simulink model "Lag_Compensator"  (R2023a)
settings: Solver=VariableStepAuto  StartTime=0.0  StopTime=30  RelTol=1e-3
settings Model: Creator=zhouwenjie  LastModifiedBy=zhouwenjie

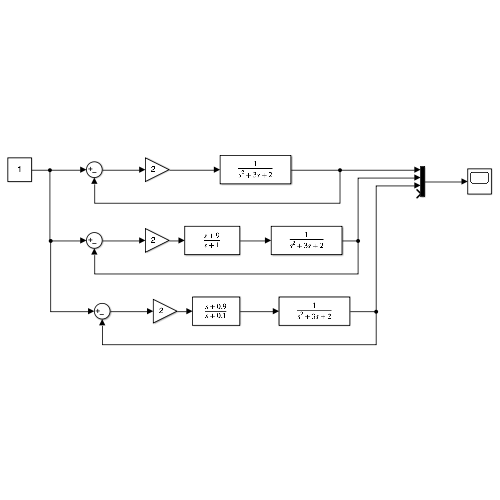
[thumbnail: Simulink's stored preview of the top-level diagram]
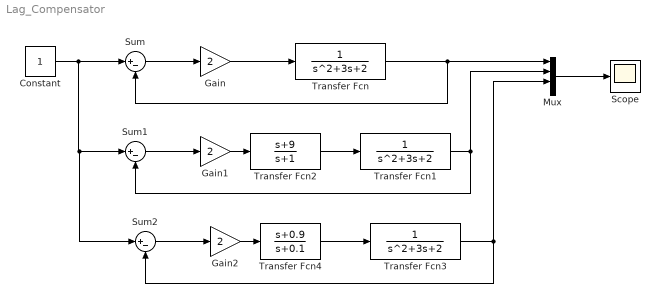
== system Lag_Compensator ==
  Constant : Constant
  Gain : Gain  Gain=2
  Gain1 : Gain  Gain=2
  Gain2 : Gain  Gain=2
  Mux : Mux
  Scope : Scope
  Sum : Sum  Inputs=|+-
  Sum1 : Sum  Inputs=|+-
  Sum2 : Sum  Inputs=|+-
  Transfer Fcn : TransferFcn  Denominator=[1 3 2]
  Transfer Fcn1 : TransferFcn  Denominator=[1 3 2]
  Transfer Fcn2 : TransferFcn  Numerator=[1 9]  Denominator=[1 1]
  Transfer Fcn3 : TransferFcn  Denominator=[1 3 2]
  Transfer Fcn4 : TransferFcn  Numerator=[1 0.9]  Denominator=[1 0.1]
  wires:
  Gain/1 -> Transfer Fcn/1
  Transfer Fcn/1 -> Sum/2, Mux/1
  Sum/1 -> Gain/1
  Mux/1 -> Scope/1
  Gain1/1 -> Transfer Fcn2/1
  Sum1/1 -> Gain1/1
  Transfer Fcn2/1 -> Transfer Fcn1/1
  Transfer Fcn1/1 -> Sum1/2, Mux/2
  Sum2/1 -> Gain2/1
  Constant/1 -> Sum2/1, Sum1/1, Sum/1
  Gain2/1 -> Transfer Fcn4/1
  Transfer Fcn4/1 -> Transfer Fcn3/1
  Transfer Fcn3/1 -> Mux/3, Sum2/2
